simulink model "Pilot_Inputs"  (R2019a)
settings: Solver=ode23t  StartTime=0.0  StopTime=10.0  MaxStep=0.001  RelTol=1e-6
model workspace (MAT data in the model file):
  A = [-0.0191  0.017  0.3839  -9.7924  -0.0008  -0.3371  0  0; 0.0136  -0.2994  0.0237  -0.5859  -0.0017  -0.0257  0.5374  0; 0.0405  -0.0026  -1.8394  0  0.0024  0.5281  0  -0.0015; 0  0  0.9985  0  0  0  0  0.0549; 0.001  -0.0017  -0.3381  0.0322  -0.0349  -0.4032  9.7777  0.1168; 0.013  0  -3.047  0  -0.229  -10.6199  0  -0.0333; 0  0  -0.0033  0  0  1  0  0.0598; 0.002  0.006  -0.5412  0  0.0039  -1.8554  0  -0.3487]
  B = [-10.3456  1.0793  0; -0.7293  0.0755  0; 27.09  -4.7239  -0.1857; 0  0  0; -1.082  -10.3713  4.7239; -27.2884  -156.4425  -1.069; 0  0  0; -4.8969  -27.9728  -12.9304]
  Cmeas = [0  0  0  1  0  0  0  0; 0  0  0  0  0  0  1  0; 0  0  0  0  0  0  0  1; 0  0  1  0  0  0  0  0; 0  0  0  0  0  1  0  0]
settings Model: DataDictionary=HeliSystemDD.sldd  FPTRunName=Active  Creator=The MathWorks Inc.  LastModifiedBy=bpotter
settings DataIOCC: LimitDataPoints=on  SaveFormat=Array  SaveOutput=off  SaveTime=off  ReturnWorkspaceOutputs=off
settings OptimizationCC: BlockReduction=off  BooleanDataType=off  UseDivisionForNetSlopeComputation=on  LifeSpan=inf
settings DebuggingCC: SaveWithParameterizedLinksMsg=none  MergeDetectMultiDrivingBlocksExec=none  SignalResolutionControl=TryResolveAllWithWarning  AllowSymbolicDim=off  PregeneratedLibrarySubsystemCodeDiagnostic=none  StrictBusMsg=ErrorOnBusTreatedAsVector  NonBusSignalsTreatedAsBus=error  SFUnexpectedBacktrackingDiag=warning  SFNoUnconditionalDefaultTransitionDiag=warning  SFExecutionAtInitializationDiag=none  ArithmeticOperatorsInVariantConditions=warning
settings HardwareCC: ProdBitPerPointer=32  ProdBitPerSizeT=32  ProdBitPerPtrDiffT=32  ProdLargestAtomicFloat=None  ProdEndianess=Unspecified  ProdWordSize=32  ProdHWDeviceType=32-bit Generic  TargetUnknown=on
settings ModelReferenceCC: PropagateSignalLabelsOutOfModel=off
settings SFSimCC: SimUseLocalCustomCode=off
settings RTWCC: RTWUseLocalCustomCode=off
settings CodeAppCC: StateflowObjectComments=on
settings GRTTargetCC: TargetLangStandard=C89/C90 (ANSI)  GeneratePreprocessorConditionals=Disable all
settings ConfigComp: CovMetricSettings=dw  CovHtmlReporting=on  CovSaveCumulativeToWorkspaceVar=on  CovSaveSingleToWorkspaceVar=on  CovExternalEMLEnable=off

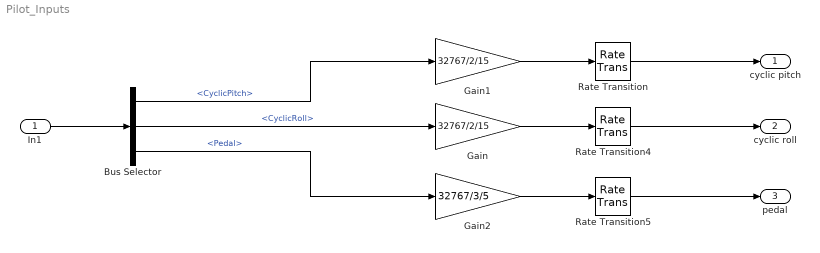
== system Pilot_Inputs ==
  In1 : Inport  OutDataTypeStr=Bus: Pilot
  Bus Selector : BusSelector  OutputSignals=CyclicPitch,CyclicRoll,Pedal
  Gain : Gain  Gain=32767/2/15  OutDataTypeStr=int16
  Gain1 : Gain  Gain=32767/2/15  OutDataTypeStr=int16
  Gain2 : Gain  Gain=32767/3/5  OutDataTypeStr=int16
  Rate Transition : RateTransition  OutPortSampleTime=0.01
  Rate Transition4 : RateTransition  OutPortSampleTime=0.01
  Rate Transition5 : RateTransition  OutPortSampleTime=0.01
  cyclic pitch : Outport  OutDataTypeStr=int16  PortDimensions=1  SampleTime=[0.01,0]
  cyclic roll : Outport  Port=2  OutDataTypeStr=int16  PortDimensions=1  SampleTime=[0.01,0]
  pedal : Outport  Port=3  OutDataTypeStr=int16  PortDimensions=1  SampleTime=[0.01,0]
  wires:
  Rate Transition/1 -> cyclic pitch/1
  Rate Transition4/1 -> cyclic roll/1
  Bus Selector/1 -> Gain1/1  "<CyclicPitch>"
  Bus Selector/3 -> Gain2/1  "<Pedal>"
  Bus Selector/2 -> Gain/1  "<CyclicRoll>"
  Gain2/1 -> Rate Transition5/1
  Gain1/1 -> Rate Transition/1
  Rate Transition5/1 -> pedal/1
  Gain/1 -> Rate Transition4/1
  In1/1 -> Bus Selector/1
